simulink model "sim"  (R2018a)
settings: Solver=VariableStepAuto  StartTime=0.0  StopTime=10.0  RelTol=1e-3
values from neighbouring files (symbols this model uses):
  b0 = 2    [matlab.mat]    (also in sys.m)
  b1 = 4    [matlab.mat]    (also in sys.m)
  b2 = 2    [matlab.mat]    (also in sys.m)
  b3 = 0    [matlab.mat]    (also in sys.m)
  k = 4    [matlab.mat]    (also in sys.m)
settings Model: Creator=daniel  LastModifiedBy=daniel

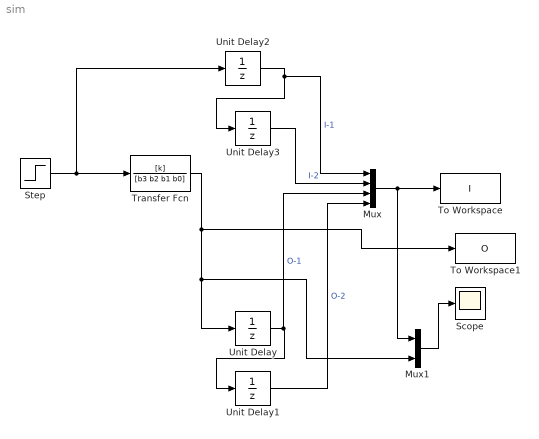
== system sim ==
  Mux : Mux
  Mux1 : Mux  Inputs=2
  Scope : Scope
  Step : Step  Time=0  SampleTime=0
  To Workspace : ToWorkspace  VariableName=I  SampleTime=-1
  To Workspace1 : ToWorkspace  VariableName=O  SampleTime=-1
  Transfer Fcn : TransferFcn  Numerator=[k]  Denominator=[b3 b2 b1 b0]
  Unit Delay{,1..3} (4 alike) : UnitDelay  SampleTime=-1
  wires:
  Transfer Fcn/1 -> To Workspace1/1, Mux1/2, Unit Delay/1
  Step/1 -> Unit Delay2/1, Transfer Fcn/1
  Unit Delay/1 -> Mux/3, Unit Delay1/1  "O-1"
  Unit Delay2/1 -> Mux/1, Unit Delay3/1  "I-1"
  Unit Delay3/1 -> Mux/2  "I-2"
  Unit Delay1/1 -> Mux/4  "O-2"
  Mux/1 -> Mux1/1, To Workspace/1
  Mux1/1 -> Scope/1
